simulink model "slexMonostaticRadarExample24a"  (R2024a)
settings: Solver=FixedStepDiscrete  StartTime=0.0  StopTime=99/paramRadar.prf  RelTol=1e-3  EnableMultiTasking=on
PreLoadFcn:
  | helperslexMonostaticRadarParam()
undefined symbols (not defined in the file or in its folder): paramRadar
libraries: phasedenvlib x4, phaseddetectlib x3, phasedtxrxlib x2, simulink x1, phasedwavlib x1, phasedmisclib x1
CloseFcn:
  | clear paramRadar
Description:
  | Monostatic Radar with One Target
settings Model: ModifiedByFormat=The MathWorks Inc.  Creator=The MathWorks, Inc.  LastModifiedBy=The MathWorks Inc.
settings SolverCC: AlgebraicLoopSolver=TrustRegion
settings DataIOCC: LimitDataPoints=on  SaveFormat=Array  SaveOutput=off  SaveTime=off  ReturnWorkspaceOutputs=off
settings OptimizationCC: ExpressionDepthLimit=2147483647  LifeSpan=inf
settings DebuggingCC: ReadBeforeWriteMsg=DisableAll  WriteAfterWriteMsg=DisableAll  WriteAfterReadMsg=DisableAll  UnderspecifiedInitializationDetection=Classic  MergeDetectMultiDrivingBlocksExec=none  SolverPrmCheckMsg=warning  MultiTaskDSMMsg=none  FcnCallInpInsideContextMsg=warning  UnconnectedInputMsg=warning  UnconnectedOutputMsg=warning  UnconnectedLineMsg=warning  AllowSymbolicDim=off  StateNameClashWarn=warning  SFUnexpectedBacktrackingDiag=warning  SFNoUnconditionalDefaultTransitionDiag=warning  SFExecutionAtInitializationDiag=none  ArithmeticOperatorsInVariantConditions=warning
settings HardwareCC: ProdBitPerPointer=32  ProdBitPerSizeT=32  ProdBitPerPtrDiffT=32  ProdLargestAtomicFloat=None  ProdIntDivRoundTo=Undefined  ProdEndianess=Unspecified  ProdWordSize=32  ProdHWDeviceType=32-bit Generic
settings ModelReferenceCC: UpdateModelReferenceTargets=IfOutOfDate  EnableRefExpFcnMdlSchedulingChecks=on  PropagateSignalLabelsOutOfModel=off
settings SFSimCC: SFSimEcho=off  SimUseLocalCustomCode=off  SimParseCustomCode=off  CustomCodeUndefinedFunction=UseInterfaceOnly
settings RTWCC: RTWUseLocalCustomCode=off  GPUComputeCapability=3.5  DLArmComputeVersion=19.05
settings CodeAppCC: StateflowObjectComments=on
settings GRTTargetCC: TargetLangStandard=C89/C90 (ANSI)  CombineOutputUpdateFcns=off  GRTInterface=on
settings ConfigComp: CovMetricSettings=dw  CovSaveCumulativeToWorkspaceVar=on  CovSaveSingleToWorkspaceVar=on  CovExternalEMLEnable=off  CovSFcnEnable=off  CovBoundaryAbsTol=1.0e-5

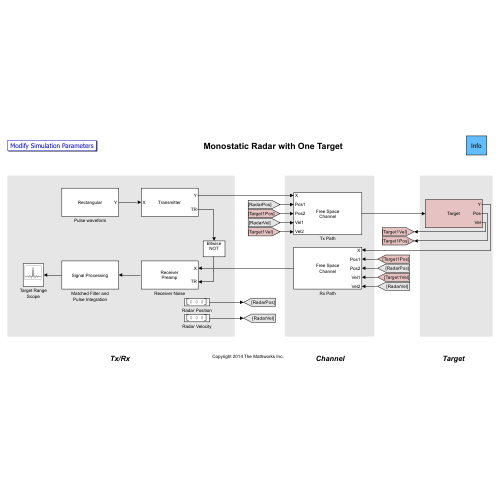
[thumbnail: Simulink's stored preview of the top-level diagram]
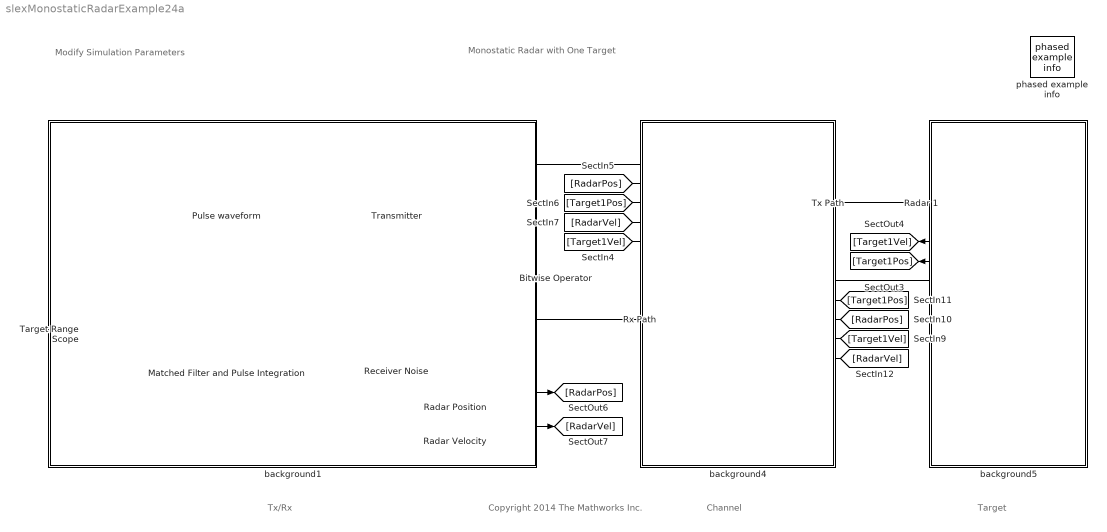
== system slexMonostaticRadarExample24a ==
  note: Monostatic Radar with One Target
  note: Tx/Rx
  note: Channel
  note: Target
  note: Modify Simulation Parameters
  note: Copyright 2014 The Mathworks Inc.
  Bitwise Operator : simulink/Logic and Bit Operations/Bitwise Operator  logicop=NOT  UseBitMask=off  BitMask=bin2dec('11011001')  BitMaskRealWorld=Stored Integer
  Matched Filter and Pulse Integration : Subsystem
      mask Display: disp('Signal Processing')
  Pulse waveform : phasedwavlib/Rectangular Waveform  SampleRate=paramRadar.fs  DurationSpecification=Pulse width  PulseWidth=1/paramRadar.pulseBw  DutyCycle=0.5  PRF=paramRadar.prf  PRFSelectionInputPort=off  SimulationTimeSource=Derive from waveform parameters  FrequencyOffsetSource=Property  FrequencyOffset=0  OutputFormat=Pulses  NumSamples=100  NumPulses=1  PRFOutputPort=off  CoefficientsOutputPort=off  SimulateUsing=Interpreted execution
  Radar 1 : Subsystem
      mask Display:
      | disp('Target')
      | port_label('output',1,'Y');
      | port_label('output',2,'Pos');
      | port_label('output',3,'Vel');
  Radar Position : Constant  Value=[ 0; 0; 0 ]  SampleTime=1/paramRadar.prf
  Radar Velocity : Constant  Value=[ 0; 0; 0 ]  SampleTime=1/paramRadar.prf
  Receiver Noise : phasedtxrxlib/Receiver Preamp  Gain=20  LossFactor=0  NoiseMethod=Noise temperature  NoiseFigure=0  ReferenceTemperature=290  SampleRateFromInputCheckbox=on  SampleRate=1e6  NoisePower=0  EnableInputPort=on  PhaseNoiseInputPort=off  SeedSource=Auto  Seed=0  SimulateUsing=Interpreted execution
  Rx Path : phasedenvlib/Free Space  PropagationSpeed=paramRadar.propSpeed  OperatingFrequency=paramRadar.fc  TwoWayPropagation=off  SampleRateFromInputCheckbox=on  SampleRate=1e6  MaximumDistanceSource=Property  MaximumDistance=10e3  MaximumNumInputSamplesSource=Auto  MaximumNumInputSamples=1000  SimulateUsing=Interpreted execution
  Target Range Scope : ArrayPlot  WindowPosition=[1.000000,41.000000,1536.000000,801.000000,]  ScopeFrameLocation=window  SampleIncrement=paramRadar.metersPerSample  XOffset=paramRadar.rangeOffset  PlotType=Line  AxesScaling=Manual  MaximizeAxes=Off  Title=Radar Return  XLabel=Range (m)  YLimits=[-4.2427e-08,1.7395e-06]
  Transmitter : phasedtxrxlib/Transmitter  InUseOutputPort=on  CoherentOnTransmit=on  PhaseNoiseOutputPort=off  SampleRate=1e6  SampleRateFromInputCheckbox=on  SimulateUsing=Interpreted execution  PeakPower=paramRadar.peakPower  GainMethod=Linear  Gain=paramRadar.txGain  LossFactor=0  OIP3=Inf  Table=[ -25, 5, -1; -10, 20, -2; 0, 27, 12; 5, 28, 12 ]  NoiseMethod=None  NoiseFigure=0  NoiseFactor=1  NoiseTemperature=0  ReferenceTemperature=290  PhaseOffset=0  SeedSource=Auto  Seed=0
  Tx Path : phasedenvlib/Free Space  PropagationSpeed=paramRadar.propSpeed  OperatingFrequency=paramRadar.fc  TwoWayPropagation=off  SampleRateFromInputCheckbox=on  SampleRate=1e6  MaximumDistanceSource=Property  MaximumDistance=10e3  MaximumNumInputSamplesSource=Auto  MaximumNumInputSamples=1000  SimulateUsing=Interpreted execution
  background1 : Subsystem  Description=Jammer
      mask Display: disp('')
  background4 : Subsystem  Description=Jammer
      mask Display: disp('')
  background5 : Subsystem  Description=Jammer
      mask Display: disp('')
  phased example info : phasedmisclib/phased example info  SystemSampleTime=-1  VariantActivationTime=update diagram  EmptyChoice=off  PassThrough=off  PassThroughVariantControl=(default)  EmptyChoiceVariantControl=(default)  AllowFlexibleInterface=on  Latency=0  AutoFrameSizeCalculation=off
  wires:
  Pulse waveform/1 -> Transmitter/1
  Receiver Noise/1 -> Matched Filter and Pulse Integration/1(In1)
  Matched Filter and Pulse Integration/1(Out1) -> Target Range Scope/1
  Transmitter/2 -> Bitwise Operator/1
  Bitwise Operator/1 -> Receiver Noise/2
  [RadarVel] -> Tx Path/4
  [Target1Pos] -> Tx Path/3
  [Target1Vel] -> Tx Path/5
  [RadarPos] -> Tx Path/2
  [Target1Vel] -> Rx Path/4
  [Target1Pos] -> Rx Path/2
  [RadarPos] -> Rx Path/3
  [RadarVel] -> Rx Path/5
  Radar 1/2(P) -> [Target1Pos]
  Tx Path/1 -> Radar 1/1(In1)
  Radar 1/1(Out1) -> Rx Path/1
  Transmitter/1 -> Tx Path/1
  Rx Path/1 -> Receiver Noise/1
  Radar Position/1 -> [RadarPos]
  Radar Velocity/1 -> [RadarVel]
  Radar 1/3(V) -> [Target1Vel]

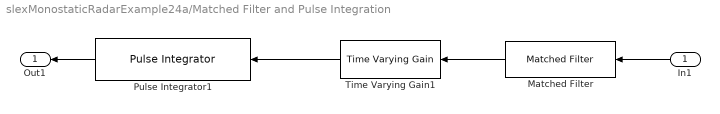
== system slexMonostaticRadarExample24a/Matched Filter and Pulse Integration ==
  In1 : Inport
  Matched Filter : phaseddetectlib/Matched Filter  CoefficientsSource=Property  Coefficients=paramRadar.matchingCoeff  SpectrumWindow=None  CustomSpectrumWindow=@hamming  SpectrumRange=[ 0, 1e5 ]  SampleRateFromInputCheckbox=on  SampleRate=1e6  SidelobeAttenuation=30  Beta=0.5  Nbar=4  GainOutputPort=off  MaximumNumInputSamplesSource=Auto  MaximumNumInputSamples=100  SimulateUsing=Interpreted execution
  Pulse Integrator1 : phaseddetectlib/Pulse Integrator  CoherentFlag=Noncoherent  N=10  V=0
  Time Varying Gain1 : phaseddetectlib/Time Varying Gain  RangeLossSource=Property  RangeLoss=paramRadar.rangeLoss  ReferenceLoss=paramRadar.referenceLoss  SimulateUsing=Interpreted execution
  Out1 : Outport  VectorParamsAs1DForOutWhenUnconnected=off
  wires:
  In1/1 -> Matched Filter/1
  Time Varying Gain1/1 -> Pulse Integrator1/1
  Matched Filter/1 -> Time Varying Gain1/1
  Pulse Integrator1/1 -> Out1/1

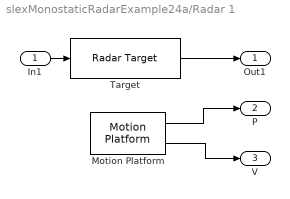
== system slexMonostaticRadarExample24a/Radar 1 ==
  In1 : Inport
  Motion Platform : phasedenvlib/Motion Platform  MotionModel=Velocity  InitialPosition=paramRadar.target1Pos  InitialVelocity=[ 0; 0; 0 ]  VelocitySource=Property  Velocity=paramRadar.target1Vel  AccelerationSource=Property  Acceleration=[0;0;0]  CustomTrajectory=[ 0, 0, 0, 0, 0, 0, 0; 1, 0, 0, 0, 0, 0, 0 ]  ScanMode=None  InitialScanAngle=0  AzimuthSpan=[ -60, 60 ]  AzimuthScanRate=10  InitialOrientationAxes=eye( 3 )  OrientationAxesOutputPort=off  ElapsedTimeSource=Auto  SampleRateFromInputCheckbox=on  SampleRate=1e6  SimulateUsing=Interpreted execution
  Target : phasedenvlib/Radar Target  EnablePolarization=off  Mode=Monostatic  MeanRCSSource=Property  ScatteringMatrixSource=Property  MeanRCS=paramRadar.target1Rcs  ScatteringMatrix=eye( 2 )  Model=Nonfluctuating  PropagationSpeed=paramRadar.propSpeed  OperatingFrequency=paramRadar.fc  SeedSource=Auto  Seed=0  SimulateUsing=Interpreted execution
  Out1 : Outport  VectorParamsAs1DForOutWhenUnconnected=off
  P : Outport  Port=2  VectorParamsAs1DForOutWhenUnconnected=off
  V : Outport  Port=3  VectorParamsAs1DForOutWhenUnconnected=off
  wires:
  In1/1 -> Target/1
  Target/1 -> Out1/1
  Motion Platform/1 -> P/1
  Motion Platform/2 -> V/1

== system slexMonostaticRadarExample24a/background1 ==

== system slexMonostaticRadarExample24a/background4 ==

== system slexMonostaticRadarExample24a/background5 ==
